simulink model "Main_C0_C3"  (R2023a)
settings: Solver=ode15s  StartTime=0.0  StopTime=1  RelTol=1e-3
model workspace (MAT data in the model file):
  C_IVD = 0.05
  E_IVD1 = 2.1
  E_IVD2 = 2.2
  E_IVD3 = 1.1
  E_IVD4 = 1.7
  E_IVD5 = 3.2
  IVD1 : object (value not decoded)
  IVD2 : object (value not decoded)
  IVD3 : object (value not decoded)
  IVD4 : object (value not decoded)
  IVD5 : object (value not decoded)
  eo_color = [1 0 0]
  io_color = [0 1 0]
  longissimus_color = [1 0 1]
  multifidus_color = [0 1 1]
  muscle_radius = 1
  psoas_color = [0 0 1]
  ra_color = [1 1 0.5]
symbols that are objects in the model workspace (value not decoded): IVD1, IVD2, IVD3, IVD4, IVD5
undefined symbols (not defined in the file or in its folder): AbdFlex, E_TLFflex, IAP_activation_AbdFlex, IAP_Pa, LeftAbdominalMuscleForce, LeftBackMuscleForce, LeftTransverse1MuscleForce, LeftTransverse2MuscleForce, RightAbdominalMuscleForce, RightBackMuscleForce, RightTransverse1MuscleForce, RightTransverse2MuscleForce, TLFflex2, X, Y, Z
libraries: nesl_utility x1235, sm_lib x960, fl_lib x6, simulink_extras x2
(part 6 of 37)

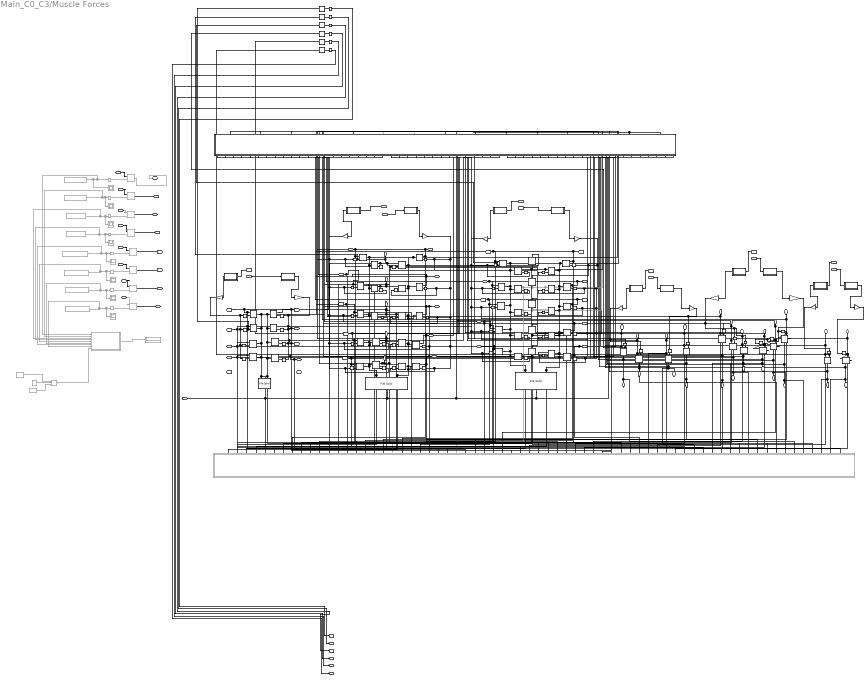
== system Main_C0_C3/Muscle Forces ==
  note: Psoas
  note: Multifidus
  note: Longissimus Thoracis
  note: External Oblique
  note: Internal Oblique
  note: Rectus Abdominus
  note: OldMuscleForces-OBSOLETE
  "Right Psoas " : Inport
  Left Psoas : Inport  Port=2
  "Right MF " : Inport  Port=3
  "Left MF " : Inport  Port=4
  "Right LongThor " : Inport  Port=5
  "Left LongThor " : Inport  Port=6
  "Right EO " : Inport  Port=7
  "Left EO " : Inport  Port=8
  "Right IO " : Inport  Port=9
  "Left IO " : Inport  Port=10
  "Right RA " : Inport  Port=11
  "Left RA " : Inport  Port=12
  Area in mm^2 : Constant  Commented=on  Value=26819
  Constant : Constant  Commented=on  Value=100000
  Display : Display  Commented=on
  Divide : Product  Commented=on  Inputs=**/
  DummyRigid Transform{,1..4} (5 alike) : sm_lib/Frames and Transforms/Rigid Transform  TranslationMethod=None  TranslationStandardOffset=0  TranslationStandardOffsetUnits=m  TranslationStandardAxis=+Z  TranslationCartesianOffset=[0 0 0]  TranslationCartesianOffsetUnits=m  TranslationROffset=0  TranslationROffsetUnits=m  TranslationZOffset=0  TranslationZOffsetUnits=m  TranslationThetaOffset=0  TranslationThetaOffsetUnits=deg  RotationMethod=None  RotationAngleUnits=deg  RotationStandardAxis=+Z  RotationAngle=0.0  RotationArbitraryAxis=[0 0 1]  FollAlignAxisA=+X  BaseAlignAxisA=+Y  FollAlignAxisB=+Y  BaseAlignAxisB=+Z  RotationSequenceAxes=FollowerAxes  RotationSequence=XYX  RotationSequenceAngles=[0 0 0]  RotationSequenceAnglesUnits=deg  RotationMatrix=[1 0 0; 0 1 0; 0 0 1]  Quaternion=[1 0 0 0]
  Gain : Gain  Gain=-0.25
  Gain1 : Gain  Gain=-0.25
  Gain10 : Gain  Gain=-1
  Gain11 : Gain  Gain=-1
  Gain{2..5} (4 alike) : Gain  Gain=-0.1
  Gain6 : Gain  Gain=-0.5
  Gain7 : Gain  Gain=-0.5
  Gain8 : Gain  Gain=-0.3333
  Gain9 : Gain  Gain=-0.3333
  IAP in Pascals : Constant  Commented=on  Value=IAP_Pa
  Internal Force{,1..7} (8 alike) : sm_lib/Forces and Torques/Internal Force  Commented=on
  Internal Force{8..12,14..16,18..69} (60 alike) : sm_lib/Forces and Torques/Internal Force
  Left Abdominal Muscle Force : Constant  Commented=on  Value=-LeftAbdominalMuscleForce
  Left Back Muscle Force : Constant  Commented=on  Value=-LeftBackMuscleForce
  Left Transverse1 Muscle Force : Constant  Commented=on  Value=-LeftTransverse1MuscleForce
  Left Transverse2 Muscle Force : Constant  Commented=on  Value=-LeftTransverse2MuscleForce
  LongissimusThoracis : sm_lib/Body Elements/File Solid  ExtGeomFileName=C:\Users\siril\OneDrive\Desktop\TIM-Control\Matlab\Simscape models\Reduced Order Model\CAD\model without nucleus\LongissimusThoracis.step  UnitType=FromFile  ExtGeomFileUnits=m  StepReaderType=HEX  ExportConvexHullGeometry=off  InertiaType=CalculateFromGeometry  Mass=1  MassUnits=g  CenterOfMass=[0 0 0]  CenterOfMassUnits=m  MomentsOfInertia=[1 1 1]  MomentsOfInertiaUnits=kg*m^2  ProductsOfInertia=[0 0 0]  ProductsOfInertiaUnits=kg*m^2  BasedOnType=Mass  Density=1000  DensityUnits=kg/m^3  DoExposeReferenceFrame=on  SerializedFrames=<Frames><Frame><Id>Frame1</Id><Value><Name>LongissimusThoracis_Right_End</Name><Origin><Source>GeometricFeature</Source><FeatureName>point 13005</FeatureName></Origin><PrimaryAxis><DefinedDirection>+Z</DefinedDirection><Source>ReferenceFrame</Source><SourceDirection>+Z</SourceDirection><FeatureName></FeatureName></PrimaryAxis><SecondaryAxis><DefinedDirection>+X</DefinedDirection><Source>ReferenceFrame</Source><SourceDirection>+X</SourceDirection><FeatureName></FeatureName></SecondaryAxis></Value></Frame><Frame><Id>Frame2</Id><Value><Name>LongissimusThoracis_Left_End</Name><Origin><Source>GeometricFeature</Source><FeatureName>point 10040</FeatureName></Origin><PrimaryAxis><DefinedDirection>+Z</DefinedDirection><Source>ReferenceFrame</Source><SourceDirection>+Z</SourceDirection><FeatureName></FeatureName></PrimaryAxis><SecondaryAxis><DefinedDirection>+X</DefinedDirection><Source>ReferenceFrame</Source><SourceDirection>+X</SourceDirection><FeatureName></FeatureName></SecondaryAxis></Value></Frame></Frames>  GraphicType=None  MarkerShape=Sphere  MarkerSize=10  GraphicVisPropType=SimpleVisualProperties  GraphicDiffuseColor=[0.5 0.5 0.5]  GraphicSpecularColor=[0.5 0.5 0.5 1.0]  GraphicAmbientColor=[0.15 0.15 0.15 1.0]  GraphicEmissiveColor=[0.0 0.0 0.0 1.0]  GraphicShininess=75  GraphicOpacity=0.5
  Multifidus : sm_lib/Body Elements/File Solid  ExtGeomFileName=C:\Users\siril\OneDrive\Desktop\TIM-Control\Matlab\Simscape models\Reduced Order Model\CAD\model without nucleus\Multifidus.step  UnitType=FromFile  ExtGeomFileUnits=m  StepReaderType=HEX  ExportConvexHullGeometry=off  InertiaType=CalculateFromGeometry  Mass=1  MassUnits=g  CenterOfMass=[0 0 0]  CenterOfMassUnits=m  MomentsOfInertia=[1 1 1]  MomentsOfInertiaUnits=kg*m^2  ProductsOfInertia=[0 0 0]  ProductsOfInertiaUnits=kg*m^2  BasedOnType=Mass  Density=1000  DensityUnits=kg/m^3  DoExposeReferenceFrame=on  SerializedFrames=<Frames><Frame><Id>Frame1</Id><Value><Name>Multifidus_Right_End</Name><Origin><Source>GeometricFeature</Source><FeatureName>segment 7296</FeatureName></Origin><PrimaryAxis><DefinedDirection>+Z</DefinedDirection><Source>ReferenceFrame</Source><SourceDirection>+Z</SourceDirection><FeatureName></FeatureName></PrimaryAxis><SecondaryAxis><DefinedDirection>+X</DefinedDirection><Source>ReferenceFrame</Source><SourceDirection>+X</SourceDirection><FeatureName></FeatureName></SecondaryAxis></Value></Frame><Frame><Id>Frame2</Id><Value><Name>Multifidus_Left_End</Name><Origin><Source>GeometricFeature</Source><FeatureName>segment 697</FeatureName></Origin><PrimaryAxis><DefinedDirection>+Z</DefinedDirection><Source>ReferenceFrame</Source><SourceDirection>+Z</SourceDirection><FeatureName></FeatureName></PrimaryAxis><SecondaryAxis><DefinedDirection>+X</DefinedDirection><Source>ReferenceFrame</Source><SourceDirection>+X</SourceDirection><FeatureName></FeatureName></SecondaryAxis></Value></Frame></Frames>  GraphicType=None  MarkerShape=Sphere  MarkerSize=10  GraphicVisPropType=SimpleVisualProperties  GraphicDiffuseColor=[0.5 0.5 0.5]  GraphicSpecularColor=[0.5 0.5 0.5 1.0]  GraphicAmbientColor=[0.15 0.15 0.15 1.0]  GraphicEmissiveColor=[0.0 0.0 0.0 1.0]  GraphicShininess=75  GraphicOpacity=0.5
  Muscle Visualization : Subsystem
  PS Gain : fl_lib/Physical Signals/Functions/PS Gain  gain=-4
  PS Gain1 : fl_lib/Physical Signals/Functions/PS Gain  gain=-10
  PS Gain2 : fl_lib/Physical Signals/Functions/PS Gain  gain=-10
  PS Gain3 : fl_lib/Physical Signals/Functions/PS Gain  gain=-2
  PS Gain4 : fl_lib/Physical Signals/Functions/PS Gain  gain=-3
  PS Gain5 : fl_lib/Physical Signals/Functions/PS Gain  gain=-1
  PS-Simulink Converter{,1..5} (6 alike) : nesl_utility/PS-Simulink Converter  PhysicalDomain=network_engine_domain  SubClassName=ps_output  LeftPortType=input  RightPortType=output  PseudoPeriodic=off  Frequencies=[]  VectorFormat=inherit  Unit=inherit  AffineConversion=off
  Psoas : sm_lib/Body Elements/File Solid  ExtGeomFileName=C:\Users\siril\OneDrive\Desktop\TIM-Control\Matlab\Simscape models\Reduced Order Model\CAD\model without nucleus\Psoas.step  UnitType=FromFile  ExtGeomFileUnits=m  StepReaderType=HEX  ExportConvexHullGeometry=off  InertiaType=CalculateFromGeometry  Mass=1  MassUnits=g  CenterOfMass=[0 0 0]  CenterOfMassUnits=m  MomentsOfInertia=[1 1 1]  MomentsOfInertiaUnits=kg*m^2  ProductsOfInertia=[0 0 0]  ProductsOfInertiaUnits=kg*m^2  BasedOnType=Mass  Density=1000  DensityUnits=kg/m^3  DoExposeReferenceFrame=on  SerializedFrames=<Frames><Frame><Id>Frame1</Id><Value><Name>Psoas_Right_End</Name><Origin><Source>GeometricFeature</Source><FeatureName>point 2042</FeatureName></Origin><PrimaryAxis><DefinedDirection>+Z</DefinedDirection><Source>ReferenceFrame</Source><SourceDirection>+Z</SourceDirection><FeatureName></FeatureName></PrimaryAxis><SecondaryAxis><DefinedDirection>+X</DefinedDirection><Source>ReferenceFrame</Source><SourceDirection>+X</SourceDirection><FeatureName></FeatureName></SecondaryAxis></Value></Frame><Frame><Id>Frame2</Id><Value><Name>Psoas_Left_End</Name><Origin><Source>GeometricFeature</Source><FeatureName>point 14414</FeatureName></Origin><PrimaryAxis><DefinedDirection>+Z</DefinedDirection><Source>ReferenceFrame</Source><SourceDirection>+Z</SourceDirection><FeatureName></FeatureName></PrimaryAxis><SecondaryAxis><DefinedDirection>+X</DefinedDirection><Source>ReferenceFrame</Source><SourceDirection>+X</SourceDirection><FeatureName></FeatureName></SecondaryAxis></Value></Frame></Frames>  GraphicType=None  MarkerShape=Sphere  MarkerSize=10  GraphicVisPropType=SimpleVisualProperties  GraphicDiffuseColor=[0.5 0.5 0.5]  GraphicSpecularColor=[0.5 0.5 0.5 1.0]  GraphicAmbientColor=[0.15 0.15 0.15 1.0]  GraphicEmissiveColor=[0.0 0.0 0.0 1.0]  GraphicShininess=75  GraphicOpacity=0.5
  Right Abdominal Muscle Force : Constant  Commented=on  Value=-RightAbdominalMuscleForce
  Right Back Muscle Force : Constant  Commented=on  Value=-RightBackMuscleForce
  Right Transverse1 Muscle Force : Constant  Commented=on  Value=-RightTransverse1MuscleForce
  Right Transverse2 Muscle Force : Constant  Commented=on  Value=-RightTransverse2MuscleForce
  Scope{1..8} (8 alike) : Scope  Commented=on
  Simulink-PS Converter{,9..12,14..16,18..69} (60 alike) : nesl_utility/Simulink-PS Converter  PhysicalDomain=network_engine_domain  SubClassName=ps_input  LeftPortType=input  RightPortType=output  PseudoPeriodic=off  Frequencies=[]  NoiseDistribution=none  NoiseParameters=[]  Unit=1  AffineConversion=off  FilteringAndDerivatives=provide  SimscapeFilterOrder=1  InputFilterTimeConstant=0.001  UdotUserProvided=0
  Simulink-PS Converter{1..8} (8 alike) : nesl_utility/Simulink-PS Converter  Commented=on  PhysicalDomain=network_engine_domain  SubClassName=ps_input  LeftPortType=input  RightPortType=output  PseudoPeriodic=off  Frequencies=[]  NoiseDistribution=none  NoiseParameters=[]  Unit=1  AffineConversion=off  FilteringAndDerivatives=provide  SimscapeFilterOrder=1  InputFilterTimeConstant=0.001  UdotUserProvided=0
  Subsystem : Subsystem
  Subsystem1 : Subsystem
  Subsystem10 : Subsystem
  Subsystem11 : Subsystem
  Subsystem2 : Subsystem
  Subsystem3 : Subsystem
  Subsystem4 : Subsystem
  Subsystem5 : Subsystem
  Subsystem6 : Subsystem
  Subsystem7 : Subsystem
  Subsystem8 : Subsystem
  Subsystem9 : Subsystem
  Sum of Square of Forces : MATLAB Function  Commented=on  TreatAsAtomicUnit=on
  Visualization : Subsystem  Commented=on
  To Right Abd Muscle on RTS : PMIOPort  Side=Right
  To Right Back Muscle on RTS : PMIOPort  Port=2  Side=Right
  To Right Tr2 Muscle on RTS : PMIOPort  Port=3  Side=Right
  To Right Tr1 Muscle on RTS : PMIOPort  Port=4  Side=Right
  To Left Abd Muscle on S1 : PMIOPort  Port=5  Side=Left
  To Right Abd Muscle on S1 : PMIOPort  Port=6  Side=Left
  To Left Back Muscle on S1 : PMIOPort  Port=7  Side=Left
  To Right Back Muscle on S1 : PMIOPort  Port=8  Side=Left
  To Right Tr2 Muscle on S1 : PMIOPort  Port=9  Side=Left
  To Right Tr1 Muscle on S1 : PMIOPort  Port=10  Side=Left
  To Left Tr2 Muscle on S1 : PMIOPort  Port=11  Side=Left
  To Left Tr1 Muscle on S1 : PMIOPort  Port=12  Side=Left
  To Left Abd Muscle on LTS : PMIOPort  Port=13  Side=Right
  To Left Back Muscle on LTS : PMIOPort  Port=14  Side=Right
  To Left Tr1 Muscle on LTS : PMIOPort  Port=15  Side=Right
  To Left Tr2 Muscle on LTS : PMIOPort  Port=16  Side=Right
  To Origin : PMIOPort  Port=17  Side=Left
  To Psoas_Right_Start_onL1 : PMIOPort  Port=18  Side=Left
  To Psoas_Left_Start_onL1 : PMIOPort  Port=19  Side=Left
  To Psoas_Right_Start_onL2 : PMIOPort  Port=20  Side=Left
  To Psoas_Right_Start_onL3 : PMIOPort  Port=21  Side=Left
  To Psoas_Right_Start_onL4 : PMIOPort  Port=22  Side=Left
  To Psoas_Right_Start_onL5 : PMIOPort  Port=23  Side=Left
  To Psoas_Left_Start_onL2 : PMIOPort  Port=24  Side=Left
  To Psoas_Left_Start_onL3 : PMIOPort  Port=25  Side=Left
  To Psoas_Left_Start_onL4 : PMIOPort  Port=26  Side=Left
  To Psoas_Left_Start_onL5 : PMIOPort  Port=27  Side=Left
  ToMuscles_SpinousProc_onL1 : PMIOPort  Port=28  Side=Left
  ToMuscles_Right_FacetJoint_onL1 : PMIOPort  Port=29  Side=Left
  ToMuscles_Left_FacetJoint_onL1 : PMIOPort  Port=30  Side=Left
  ToMuscles_Right_FacetJoint_onL2 : PMIOPort  Port=31  Side=Left
  ToMuscles_Left_FacetJoint_onL2 : PMIOPort  Port=32  Side=Left
  ToMuscles_SpinousProc_onL2 : PMIOPort  Port=33  Side=Left
  ToMuscles_Right_FacetJoint_onL3 : PMIOPort  Port=34  Side=Left
  ToMuscles_SpinousProc_onL3 : PMIOPort  Port=35  Side=Left
  ToMuscles_Left_FacetJoint_onL3 : PMIOPort  Port=36  Side=Left
  ToMuscles_Right_FacetJoint_onL4 : PMIOPort  Port=37  Side=Left
  ToMuscles_SpinousProc_onL4 : PMIOPort  Port=38  Side=Left
  ToMuscles_Left_FacetJoint_onL4 : PMIOPort  Port=39  Side=Left
  ToMuscles_Right_FacetJoint_onL5 : PMIOPort  Port=40  Side=Left
  ToMuscles_SpinousProc_onL5 : PMIOPort  Port=41  Side=Left
  ToMuscles_Left_FacetJoint_onL5 : PMIOPort  Port=42  Side=Left
  ToMuscles_Right_TransvProc_onL1 : PMIOPort  Port=43  Side=Left
  ToMuscles_Left_TransvProc_onL1 : PMIOPort  Port=44  Side=Left
  ToMuscles_Right_TransvProc_onL2 : PMIOPort  Port=45  Side=Left
  ToMuscles_Right_TransvProc_onL3 : PMIOPort  Port=46  Side=Left
  ToMuscles_Right_TransvProc_onL4 : PMIOPort  Port=47  Side=Left
  ToMuscles_Right_TransvProc_onL5 : PMIOPort  Port=48  Side=Left
  ToMuscles_Left_TransvProc_onL2 : PMIOPort  Port=49  Side=Left
  ToMuscles_Left_TransvProc_onL3 : PMIOPort  Port=50  Side=Left
  ToMuscles_Left_TransvProc_onL4 : PMIOPort  Port=51  Side=Left
  ToMuscles_Left_TransvProc_onL5 : PMIOPort  Port=52  Side=Left
  E01_Right_End_onTSpine : PMIOPort  Port=53  Side=Left
  E01_Left_End_onTSpine : PMIOPort  Port=54  Side=Left
  E02_Right_End_onTSpine : PMIOPort  Port=55  Side=Left
  E02_Left_End_onTSpine : PMIOPort  Port=56  Side=Left
  E01_Right_Start_onS1 : PMIOPort  Port=57  Side=Left
  E02_Right_Start_onS1 : PMIOPort  Port=58  Side=Left
  E01_Left_Start_onS1 : PMIOPort  Port=59  Side=Left
  E02_Left_Start_onS1 : PMIOPort  Port=60  Side=Left
  IO1_Right_End_onTSpine : PMIOPort  Port=61  Side=Left
  IO2_Right_End_onTSpine : PMIOPort  Port=62  Side=Left
  IO3_Right_End_onTSpine : PMIOPort  Port=63  Side=Left
  IO1_Left_End_onTSpine : PMIOPort  Port=64  Side=Left
  IO2_Left_End_onTSpine : PMIOPort  Port=65  Side=Left
  IO3_Left_End_onTSpine : PMIOPort  Port=66  Side=Left
  IO1_Right_Start_onS1 : PMIOPort  Port=67  Side=Left
  IO2_Right_Start_onS1 : PMIOPort  Port=68  Side=Left
  IO3_Right_Start_onS1 : PMIOPort  Port=69  Side=Left
  IO1_Left_Start_onS1 : PMIOPort  Port=70  Side=Left
  IO2_Left_Start_onS1 : PMIOPort  Port=71  Side=Left
  IO3_Left_Start_onS1 : PMIOPort  Port=72  Side=Left
  RA_Right_End_onTSpine : PMIOPort  Port=73  Side=Left
  RA_Left_End_onTSpine : PMIOPort  Port=74  Side=Left
  RA_Right_Start_onS1 : PMIOPort  Port=75  Side=Left
  RA_Left_Start_onS1 : PMIOPort  Port=76  Side=Left
  Left Psoas force : Outport
  Left MF force : Outport  Port=2
  Left LongThor force : Outport  Port=3
  Left EO force : Outport  Port=4
  Left IO force : Outport  Port=5
  Left RA force : Outport  Port=6
  wires:
  "Left RA "/1 -> Subsystem11/1(Muslce force)
  "Right RA "/1 -> Subsystem10/1(Muslce force)
  "Left IO "/1 -> Subsystem9/1(Muslce force)
  "Right IO "/1 -> Subsystem8/1(Muslce force)
  "Left EO "/1 -> Subsystem7/1(Muslce force)
  "Right EO "/1 -> Subsystem6/1(Muslce force)
  "Left LongThor "/1 -> Subsystem5/1(Muslce force)
  "Right LongThor "/1 -> Subsystem4/1(Muslce force)
  "Left MF "/1 -> Subsystem3/1(Muslce force)
  "Right MF "/1 -> Subsystem2/1(Muslce force)
  Left Psoas/1 -> Subsystem1/1(Muslce force)
  "Right Psoas "/1 -> Subsystem/1(Muslce force)
  PS-Simulink Converter5/1 -> Left RA force/1  "Left RA"
  PS-Simulink Converter4/1 -> Left IO force/1  "Left IO"
  PS-Simulink Converter3/1 -> Left EO force/1  "Left EO"
  PS-Simulink Converter2/1 -> Left LongThor force/1  "Left LongThor"
  PS-Simulink Converter1/1 -> Left MF force/1  "Left MF"
  PS-Simulink Converter/1 -> Left Psoas force/1  "Left Psoas"
  Subsystem11/1(Out1) -> Gain11/1
  Subsystem10/1(Out1) -> Gain10/1
  Subsystem9/1(Out1) -> Gain9/1
  Subsystem8/1(Out1) -> Gain8/1
  Subsystem7/1(Out1) -> Gain6/1
  Subsystem6/1(Out1) -> Gain7/1
  Subsystem5/1(Out1) -> Gain4/1
  Subsystem4/1(Out1) -> Gain5/1
  Subsystem3/1(Out1) -> Gain3/1
  Subsystem2/1(Out1) -> Gain2/1
  Gain11/1 -> Simulink-PS Converter69/1
  Gain10/1 -> Simulink-PS Converter68/1
  Subsystem1/1(Out1) -> Gain1/1
  Subsystem/1(Out1) -> Gain/1
  Gain9/1 -> Simulink-PS Converter67/1, Simulink-PS Converter66/1, Simulink-PS Converter65/1
  Gain8/1 -> Simulink-PS Converter64/1, Simulink-PS Converter63/1, Simulink-PS Converter62/1
  Gain7/1 -> Simulink-PS Converter59/1, Simulink-PS Converter58/1
  Gain6/1 -> Simulink-PS Converter60/1, Simulink-PS Converter61/1
  Gain4/1 -> Simulink-PS Converter40/1, Simulink-PS Converter41/1, Simulink-PS Converter44/1, Simulink-PS Converter45/1, Simulink-PS Converter49/1, Simulink-PS Converter47/1, Simulink-PS Converter52/1, Simulink-PS Converter51/1, Simulink-PS Converter56/1, Simulink-PS Converter55/1
  Gain5/1 -> Simulink-PS Converter42/1, Simulink-PS Converter43/1, Simulink-PS Converter46/1, Simulink-PS Converter48/1, Simulink-PS Converter50/1, Simulink-PS Converter53/1, Simulink-PS Converter54/1, Simulink-PS Converter57/1, Simulink-PS Converter38/1, Simulink-PS Converter39/1
  Gain3/1 -> Simulink-PS Converter25/1, Simulink-PS Converter24/1, Simulink-PS Converter29/1, Simulink-PS Converter28/1, Simulink-PS Converter33/1, Simulink-PS Converter32/1, Simulink-PS Converter37/1, Simulink-PS Converter36/1, Simulink-PS Converter19/1, Simulink-PS Converter21/1
  Gain2/1 -> Simulink-PS Converter26/1, Simulink-PS Converter27/1, Simulink-PS Converter30/1, Simulink-PS Converter31/1, Simulink-PS Converter34/1, Simulink-PS Converter35/1, Simulink-PS Converter22/1, Simulink-PS Converter23/1, Simulink-PS Converter20/1, Simulink-PS Converter18/1
  Gain1/1 -> Simulink-PS Converter16/1, Simulink-PS Converter15/1, Simulink-PS Converter14/1, Simulink-PS Converter9/1
  Gain/1 -> Simulink-PS Converter/1, Simulink-PS Converter10/1, Simulink-PS Converter11/1, Simulink-PS Converter12/1
  Divide/1 -> Sum of Square of Forces/9(IAP)
  Area in mm^2/1 -> Divide/2
  Constant/1 -> Divide/3
  IAP in Pascals/1 -> Divide/1
  Left Transverse2 Muscle Force/1 -> Simulink-PS Converter8/1, Scope8/1, Sum of Square of Forces/8(F8)  "LeftTransverse2MuscleForce"
  Right Transverse1 Muscle Force/1 -> Sum of Square of Forces/7(F7), Simulink-PS Converter5/1, Scope5/1  "RightTransverse1MuscleForce"
  Left Transverse1 Muscle Force/1 -> Sum of Square of Forces/6(F6), Simulink-PS Converter7/1, Scope7/1  "LeftTransverse1MuscleForce"
  Right Transverse2 Muscle Force/1 -> Simulink-PS Converter6/1, Scope6/1, Sum of Square of Forces/5(F5)  "RightTransverse2MuscleForce"
  Left Back Muscle Force/1 -> Simulink-PS Converter4/1, Scope4/1, Sum of Square of Forces/4(F4)  "LeftBackMuscleForce"
  Right Back Muscle Force/1 -> Sum of Square of Forces/3(F3), Simulink-PS Converter3/1, Scope3/1  "RightBackMuscleForce"
  Left Abdominal Muscle Force/1 -> Sum of Square of Forces/2(F2), Simulink-PS Converter2/1, Scope2/1  "LeftAbdominalMuscleForce"
  Right Abdominal Muscle Force/1 -> Scope1/1, Simulink-PS Converter1/1, Sum of Square of Forces/1(F1)  "RightAbdominalMuscleForce"
  Sum of Square of Forces/1(SumofSquareofForces) -> Display/1  "SumofSquareofForces"
  connections:
  PS-Simulink Converter5/LConn1 -- PS Gain5/RConn1
  PS-Simulink Converter4/LConn1 -- PS Gain4/RConn1
  PS-Simulink Converter3/LConn1 -- PS Gain3/RConn1
  PS-Simulink Converter2/LConn1 -- PS Gain2/RConn1
  PS-Simulink Converter1/LConn1 -- PS Gain1/RConn1
  PS-Simulink Converter/LConn1 -- PS Gain/RConn1
  Muscle Visualization/RConn56 -- Psoas/RConn1 -- To Origin/RConn1 -- Multifidus/RConn1 -- Muscle Visualization/LConn14 -- Muscle Visualization/LConn15 -- LongissimusThoracis/RConn1
  Multifidus/LConn1 -- Visualization/LConn2 -- Internal Force34/RConn1 -- Internal Force35/RConn1 -- Internal Force30/RConn1 -- Internal Force27/RConn1 -- Internal Force26/RConn1 -- Internal Force23/RConn1 -- Internal Force22/RConn1 -- Internal Force19/RConn1 -- Internal Force18/RConn1 -- Muscle Visualization/LConn1 -- Internal Force31/RConn1
  ToMuscles_SpinousProc_onL1/RConn1 -- Muscle Visualization/RConn5 -- Internal Force20/LConn1 -- DummyRigid Transform/LConn1 -- Visualization/LConn12 -- Internal Force19/LConn1
  ToMuscles_Left_FacetJoint_onL4/RConn1 -- Muscle Visualization/RConn29 -- Internal Force33/LConn1 -- Visualization/LConn37
  IO3_Left_End_onTSpine/RConn1 -- Muscle Visualization/RConn19 -- Visualization/LConn28 -- Internal Force67/LConn1
  RA_Right_End_onTSpine/RConn1 -- Muscle Visualization/RConn36 -- Visualization/LConn48 -- Internal Force68/LConn1
  DummyRigid Transform3/RConn1 -- Visualization/LConn38 -- Internal Force51/LConn1 -- Muscle Visualization/LConn10 -- Internal Force53/LConn1
  LongissimusThoracis/LConn1 -- Visualization/LConn3 -- Internal Force57/RConn1 -- Internal Force54/RConn1 -- Internal Force39/RConn1 -- Muscle Visualization/LConn3 -- Internal Force38/RConn1 -- Internal Force42/RConn1 -- Internal Force43/RConn1 -- Internal Force46/RConn1 -- Internal Force48/RConn1 -- Internal Force50/RConn1 -- Internal Force53/RConn1
  Internal Force69/RConn1 -- Muscle Visualization/RConn54 -- Visualization/LConn67 -- RA_Left_Start_onS1/RConn1
  Internal Force68/RConn1 -- Muscle Visualization/RConn55 -- Visualization/LConn66 -- RA_Right_Start_onS1/RConn1
  RA_Left_End_onTSpine/RConn1 -- Muscle Visualization/RConn32 -- Visualization/LConn50 -- Internal Force69/LConn1
  Simulink-PS Converter69/RConn1 -- Internal Force69/LConn2
  Internal Force68/LConn2 -- PS Gain5/LConn1 -- Simulink-PS Converter68/RConn1
  Internal Force67/RConn1 -- Muscle Visualization/RConn51 -- Visualization/LConn64 -- IO3_Left_Start_onS1/RConn1
  IO2_Left_End_onTSpine/RConn1 -- Muscle Visualization/RConn25 -- Visualization/LConn31 -- Internal Force66/LConn1
  Internal Force66/RConn1 -- Muscle Visualization/RConn49 -- Visualization/LConn62 -- IO2_Left_Start_onS1/RConn1
  IO1_Left_End_onTSpine/RConn1 -- Muscle Visualization/RConn30 -- Visualization/LConn40 -- Internal Force65/LConn1
  Internal Force65/RConn1 -- Muscle Visualization/RConn47 -- Visualization/LConn56 -- IO1_Left_Start_onS1/RConn1
  IO3_Right_End_onTSpine/RConn1 -- Muscle Visualization/RConn18 -- Visualization/LConn34 -- Internal Force64/LConn1
  Internal Force64/RConn1 -- Muscle Visualization/RConn40 -- Visualization/LConn68 -- IO3_Right_Start_onS1/RConn1
  IO2_Right_End_onTSpine/RConn1 -- Muscle Visualization/RConn24 -- Visualization/LConn36 -- Internal Force63/LConn1
  Internal Force63/RConn1 -- Muscle Visualization/RConn45 -- Visualization/LConn58 -- IO2_Right_Start_onS1/RConn1
  Internal Force62/RConn1 -- Muscle Visualization/RConn43 -- Visualization/LConn54 -- IO1_Right_Start_onS1/RConn1
  Internal Force62/LConn1 -- Visualization/LConn41 -- Muscle Visualization/RConn31 -- IO1_Right_End_onTSpine/RConn1
  Simulink-PS Converter67/RConn1 -- Internal Force67/LConn2
  Simulink-PS Converter65/RConn1 -- Internal Force65/LConn2
  Simulink-PS Converter66/RConn1 -- Internal Force66/LConn2
  Internal Force64/LConn2 -- PS Gain4/LConn1 -- Simulink-PS Converter64/RConn1
  Simulink-PS Converter63/RConn1 -- Internal Force63/LConn2
  Simulink-PS Converter62/RConn1 -- Internal Force62/LConn2
  E02_Left_End_onTSpine/RConn1 -- Muscle Visualization/RConn27 -- Visualization/LConn39 -- Internal Force61/LConn1
  E02_Left_Start_onS1/RConn1 -- Visualization/LConn18 -- Muscle Visualization/RConn50 -- Internal Force61/RConn1
  E01_Left_End_onTSpine/RConn1 -- Muscle Visualization/RConn35 -- Visualization/LConn47 -- Internal Force60/LConn1
  Internal Force60/RConn1 -- Muscle Visualization/RConn52 -- Visualization/LConn60 -- E01_Left_Start_onS1/RConn1
  Internal Force58/LConn1 -- Visualization/LConn49 -- Muscle Visualization/RConn34 -- E01_Right_End_onTSpine/RConn1
  E02_Right_Start_onS1/RConn1 -- Visualization/LConn63 -- Muscle Visualization/RConn48 -- Internal Force59/RConn1
  Internal Force59/LConn1 -- Visualization/LConn42 -- Muscle Visualization/RConn26 -- E02_Right_End_onTSpine/RConn1
  E01_Right_Start_onS1/RConn1 -- Visualization/LConn61 -- Muscle Visualization/RConn53 -- Internal Force58/RConn1
  Simulink-PS Converter61/RConn1 -- Internal Force61/LConn2
  Simulink-PS Converter60/RConn1 -- Internal Force60/LConn2
  Internal Force59/LConn2 -- PS Gain3/LConn1 -- Simulink-PS Converter59/RConn1
  Simulink-PS Converter58/RConn1 -- Internal Force58/LConn2
  ToMuscles_Left_TransvProc_onL5/RConn1 -- Muscle Visualization/RConn39 -- Visualization/LConn46 -- Internal Force56/LConn1
  DummyRigid Transform4/RConn1 -- Visualization/LConn52 -- Internal Force55/LConn1 -- Muscle Visualization/LConn12 -- Internal Force57/LConn1
  Internal Force54/LConn1 -- Visualization/LConn45 -- Muscle Visualization/RConn38 -- ToMuscles_Right_TransvProc_onL5/RConn1
  Simulink-PS Converter57/RConn1 -- Internal Force57/LConn2
  Simulink-PS Converter56/RConn1 -- Internal Force56/LConn2
  Simulink-PS Converter55/RConn1 -- Internal Force55/LConn2
  Simulink-PS Converter54/RConn1 -- Internal Force54/LConn2
  ToMuscles_Left_TransvProc_onL4/RConn1 -- Muscle Visualization/RConn21 -- Visualization/LConn29 -- Internal Force52/LConn1
  Internal Force50/LConn1 -- Visualization/LConn30 -- Muscle Visualization/RConn20 -- ToMuscles_Right_TransvProc_onL4/RConn1
  Simulink-PS Converter53/RConn1 -- Internal Force53/LConn2
  Simulink-PS Converter52/RConn1 -- Internal Force52/LConn2
  Simulink-PS Converter51/RConn1 -- Internal Force51/LConn2
  Simulink-PS Converter50/RConn1 -- Internal Force50/LConn2
  ToMuscles_Left_TransvProc_onL3/RConn1 -- Muscle Visualization/RConn12 -- Visualization/LConn20 -- Internal Force49/LConn1
  Visualization/LConn26 -- DummyRigid Transform2/RConn1 -- Internal Force47/LConn1 -- Muscle Visualization/LConn7 -- Internal Force48/LConn1
  Internal Force46/LConn1 -- Visualization/LConn22 -- Muscle Visualization/RConn11 -- ToMuscles_Right_TransvProc_onL3/RConn1
  Simulink-PS Converter49/RConn1 -- Internal Force49/LConn2
  Simulink-PS Converter48/RConn1 -- Internal Force48/LConn2
  Simulink-PS Converter47/RConn1 -- Internal Force47/LConn2
  Simulink-PS Converter46/RConn1 -- Internal Force46/LConn2
  ToMuscles_Left_TransvProc_onL2/RConn1 -- Muscle Visualization/RConn9 -- Visualization/LConn16 -- Internal Force44/LConn1
  Visualization/LConn19 -- DummyRigid Transform1/RConn1 -- Internal Force45/LConn1 -- Muscle Visualization/LConn6 -- Internal Force43/LConn1
  Internal Force42/LConn1 -- Visualization/LConn15 -- Muscle Visualization/RConn8 -- ToMuscles_Right_TransvProc_onL2/RConn1
  Simulink-PS Converter45/RConn1 -- Internal Force45/LConn2
  Simulink-PS Converter44/RConn1 -- Internal Force44/LConn2
  Simulink-PS Converter43/RConn1 -- Internal Force43/LConn2
  Simulink-PS Converter42/RConn1 -- Internal Force42/LConn2
  Internal Force39/LConn1 -- Visualization/LConn7 -- Internal Force41/LConn1 -- Muscle Visualization/LConn5 -- DummyRigid Transform/RConn1
  LongissimusThoracis/LConn2 -- Visualization/LConn4 -- Internal Force56/RConn1 -- Internal Force55/RConn1 -- Internal Force51/RConn1 -- Internal Force52/RConn1 -- Internal Force47/RConn1 -- Internal Force49/RConn1 -- Internal Force45/RConn1 -- Internal Force44/RConn1 -- Internal Force41/RConn1 -- Muscle Visualization/LConn4 -- Internal Force40/RConn1
  Internal Force40/LConn1 -- Visualization/LConn9 -- Muscle Visualization/RConn4 -- ToMuscles_Left_TransvProc_onL1/RConn1
  Internal Force38/LConn1 -- Visualization/LConn11 -- Muscle Visualization/RConn3 -- ToMuscles_Right_TransvProc_onL1/RConn1
  Simulink-PS Converter41/RConn1 -- Internal Force41/LConn2
  Simulink-PS Converter40/RConn1 -- Internal Force40/LConn2
  Simulink-PS Converter39/RConn1 -- Internal Force39/LConn2
  Internal Force38/LConn2 -- PS Gain2/LConn1 -- Simulink-PS Converter38/RConn1
  ToMuscles_SpinousProc_onL5/RConn1 -- DummyRigid Transform4/LConn1 -- Visualization/LConn57 -- Internal Force36/LConn1 -- Muscle Visualization/LConn13 -- Internal Force35/LConn1
  Internal Force37/LConn1 -- Visualization/LConn59 -- Muscle Visualization/RConn42 -- ToMuscles_Left_FacetJoint_onL5/RConn1
  Internal Force34/LConn1 -- Visualization/LConn53 -- Muscle Visualization/RConn46 -- ToMuscles_Right_FacetJoint_onL5/RConn1
  Simulink-PS Converter37/RConn1 -- Internal Force37/LConn2
  Simulink-PS Converter36/RConn1 -- Internal Force36/LConn2
  Simulink-PS Converter35/RConn1 -- Internal Force35/LConn2
  Simulink-PS Converter34/RConn1 -- Internal Force34/LConn2
  ToMuscles_SpinousProc_onL4/RConn1 -- Muscle Visualization/LConn11 -- DummyRigid Transform3/LConn1 -- Visualization/LConn6 -- Internal Force32/LConn1 -- Internal Force31/LConn1
  Internal Force30/LConn1 -- Visualization/LConn35 -- Muscle Visualization/RConn28 -- ToMuscles_Right_FacetJoint_onL4/RConn1
  Simulink-PS Converter33/RConn1 -- Internal Force33/LConn2
  Simulink-PS Converter32/RConn1 -- Internal Force32/LConn2
  Simulink-PS Converter31/RConn1 -- Internal Force31/LConn2
  Simulink-PS Converter30/RConn1 -- Internal Force30/LConn2
  ToMuscles_Left_FacetJoint_onL3/RConn1 -- Visualization/LConn23 -- Muscle Visualization/RConn14 -- Internal Force29/LConn1
  ToMuscles_SpinousProc_onL3/RConn1 -- Muscle Visualization/RConn15 -- DummyRigid Transform2/LConn1 -- Internal Force28/LConn1 -- Visualization/LConn27 -- Internal Force27/LConn1
  Internal Force26/LConn1 -- Visualization/LConn21 -- Muscle Visualization/RConn13 -- ToMuscles_Right_FacetJoint_onL3/RConn1
  Simulink-PS Converter29/RConn1 -- Internal Force29/LConn2
  Simulink-PS Converter28/RConn1 -- Internal Force28/LConn2
  Simulink-PS Converter27/RConn1 -- Internal Force27/LConn2
  Simulink-PS Converter26/RConn1 -- Internal Force26/LConn2
  Internal Force25/LConn1 -- Visualization/LConn14 -- Muscle Visualization/RConn7 -- ToMuscles_Left_FacetJoint_onL2/RConn1
  Internal Force23/LConn1 -- Visualization/LConn17 -- Internal Force24/LConn1 -- Muscle Visualization/RConn10 -- DummyRigid Transform1/LConn1 -- ToMuscles_SpinousProc_onL2/RConn1
  Internal Force22/LConn1 -- Visualization/LConn13 -- Muscle Visualization/RConn6 -- ToMuscles_Right_FacetJoint_onL2/RConn1
  Simulink-PS Converter25/RConn1 -- Internal Force25/LConn2
  Simulink-PS Converter24/RConn1 -- Internal Force24/LConn2
  Simulink-PS Converter23/RConn1 -- Internal Force23/LConn2
  Simulink-PS Converter22/RConn1 -- Internal Force22/LConn2
  Internal Force18/LConn2 -- PS Gain1/LConn1 -- Simulink-PS Converter18/RConn1
  Simulink-PS Converter19/RConn1 -- Internal Force21/LConn2
  Simulink-PS Converter20/RConn1 -- Internal Force19/LConn2
  Simulink-PS Converter21/RConn1 -- Internal Force20/LConn2
  Internal Force28/RConn1 -- Internal Force36/RConn1 -- Multifidus/LConn2 -- Visualization/LConn1 -- Internal Force37/RConn1 -- Internal Force33/RConn1 -- Internal Force32/RConn1 -- Internal Force29/RConn1 -- Internal Force24/RConn1 -- Internal Force25/RConn1 -- Internal Force20/RConn1 -- Muscle Visualization/LConn2 -- Internal Force21/RConn1
  ToMuscles_Left_FacetJoint_onL1/RConn1 -- Muscle Visualization/RConn2 -- Visualization/LConn8 -- Internal Force21/LConn1
  ToMuscles_Right_FacetJoint_onL1/RConn1 -- Muscle Visualization/RConn1 -- Visualization/LConn10 -- Internal Force18/LConn1
  Internal Force16/LConn1 -- Muscle Visualization/RConn41 -- Visualization/LConn55 -- To Psoas_Left_Start_onL4/RConn1
  Internal Force15/LConn1 -- Muscle Visualization/RConn33 -- Visualization/LConn43 -- To Psoas_Left_Start_onL3/RConn1
  Internal Force14/LConn1 -- Muscle Visualization/RConn23 -- Visualization/LConn32 -- To Psoas_Left_Start_onL2/RConn1
  Simulink-PS Converter16/RConn1 -- Internal Force16/LConn2
  Simulink-PS Converter15/RConn1 -- Internal Force15/LConn2
  Simulink-PS Converter14/RConn1 -- Internal Force14/LConn2
  Simulink-PS Converter12/RConn1 -- Internal Force12/LConn2
  Simulink-PS Converter11/RConn1 -- Internal Force11/LConn2
  Internal Force10/LConn2 -- PS Gain/LConn1 -- Simulink-PS Converter10/RConn1
  Internal Force12/LConn1 -- Visualization/LConn51 -- Muscle Visualization/RConn44 -- To Psoas_Right_Start_onL4/RConn1
  Internal Force11/LConn1 -- Visualization/LConn44 -- Muscle Visualization/RConn37 -- To Psoas_Right_Start_onL3/RConn1
  Internal Force10/LConn1 -- Muscle Visualization/RConn22 -- Visualization/LConn33 -- To Psoas_Right_Start_onL2/RConn1
  Simulink-PS Converter9/RConn1 -- Internal Force9/LConn2
  Simulink-PS Converter/RConn1 -- Internal Force8/LConn2
  Psoas/LConn2 -- Visualization/LConn65 -- Internal Force16/RConn1 -- Internal Force15/RConn1 -- Internal Force14/RConn1 -- Muscle Visualization/LConn9 -- Internal Force9/RConn1
  To Psoas_Left_Start_onL1/RConn1 -- Visualization/LConn25 -- Muscle Visualization/RConn17 -- Internal Force9/LConn1
  Internal Force10/RConn1 -- Internal Force11/RConn1 -- Internal Force12/RConn1 -- Psoas/LConn1 -- Visualization/LConn5 -- Muscle Visualization/LConn8 -- Internal Force8/RConn1
  Internal Force8/LConn1 -- Visualization/LConn24 -- Muscle Visualization/RConn16 -- To Psoas_Right_Start_onL1/RConn1
  Internal Force/RConn1 -- To Right Abd Muscle on RTS/RConn1
  To Left Abd Muscle on S1/RConn1 -- Internal Force1/LConn1
  To Left Tr2 Muscle on LTS/RConn1 -- Internal Force7/RConn1
  To Left Tr1 Muscle on S1/RConn1 -- Internal Force6/LConn1
  To Right Tr1 Muscle on S1/RConn1 -- Internal Force4/LConn1
  To Right Tr2 Muscle on S1/RConn1 -- Internal Force5/LConn1
  To Left Back Muscle on LTS/RConn1 -- Internal Force3/RConn1
  Simulink-PS Converter7/RConn1 -- Internal Force6/LConn2
  Simulink-PS Converter5/RConn1 -- Internal Force4/LConn2
  Simulink-PS Converter4/RConn1 -- Internal Force3/LConn2
  To Right Abd Muscle on S1/RConn1 -- Internal Force/LConn1
  Simulink-PS Converter3/RConn1 -- Internal Force2/LConn2
  Simulink-PS Converter2/RConn1 -- Internal Force1/LConn2
  To Left Abd Muscle on LTS/RConn1 -- Internal Force1/RConn1
  To Right Back Muscle on RTS/RConn1 -- Internal Force2/RConn1
  Internal Force7/LConn1 -- To Left Tr2 Muscle on S1/RConn1
  To Right Tr2 Muscle on RTS/RConn1 -- Internal Force5/RConn1
  To Left Tr1 Muscle on LTS/RConn1 -- Internal Force6/RConn1
  Simulink-PS Converter1/RConn1 -- Internal Force/LConn2
  Simulink-PS Converter6/RConn1 -- Internal Force5/LConn2
  To Right Tr1 Muscle on RTS/RConn1 -- Internal Force4/RConn1
  Simulink-PS Converter8/RConn1 -- Internal Force7/LConn2
  To Left Back Muscle on S1/RConn1 -- Internal Force3/LConn1
  Internal Force2/LConn1 -- To Right Back Muscle on S1/RConn1

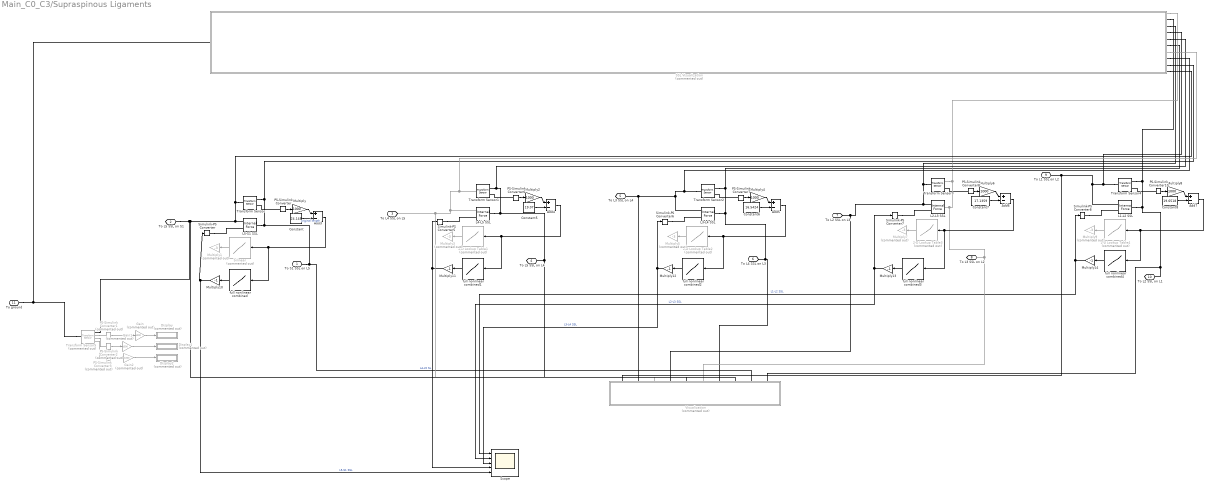
== system Main_C0_C3/Supraspinous Ligaments ==
  2-D Lookup Table1 : Lookup_n-D  Commented=on  NumberOfTableDimensions=1  BreakpointsForDimension1=[0;0.223;3.345;4.906;6.467]  BreakpointsForDimension2=[1:3]  Table=[0;0;8.4;21;84]  InternalRulePriority=Speed  RndMeth=Simplest
  2-D Lookup Table2 : Lookup_n-D  Commented=on  NumberOfTableDimensions=1  BreakpointsForDimension1=[0;0.194;2.91;4.268;5.626]  BreakpointsForDimension2=[1:3]  Table=[0;0;8.4;21;84]  InternalRulePriority=Speed  RndMeth=Simplest
  2-D Lookup Table3 : Lookup_n-D  Commented=on  NumberOfTableDimensions=1  BreakpointsForDimension1=[0;0.268;4.02;5.896;7.772]  BreakpointsForDimension2=[1:3]  Table=[0;0;8.4;21;84]  InternalRulePriority=Speed  RndMeth=Simplest
  2-D Lookup Table4 : Lookup_n-D  Commented=on  NumberOfTableDimensions=1  BreakpointsForDimension1=[0;0.223;3.345;4.906;6.467]  BreakpointsForDimension2=[1:3]  Table=[0;0;8.4;21;84]  InternalRulePriority=Speed  RndMeth=Simplest
  Add{3..7} (5 alike) : Sum  Inputs=+-
  Constant : Constant  Value=24.148
  Constant5 : Constant  Value=19.07
  Constant6 : Constant  Value=16.5424
  Constant7 : Constant  Value=17.1359
  Constant8 : Constant  Value=19.6518
  Display : Display  Commented=on
  Display1 : Display  Commented=on
  Display2 : Display  Commented=on
  Gain : Gain  Commented=on  Gain=1000
  Gain1 : Gain  Commented=on  Gain=1000
  Gain2 : Gain  Commented=on  Gain=1000
  L1-L2 SSL : sm_lib/Forces and Torques/Internal Force
  L2-L3 SSL : sm_lib/Forces and Torques/Internal Force
  L3-L4 SSL : sm_lib/Forces and Torques/Internal Force
  L4-L5 SSL : sm_lib/Forces and Torques/Internal Force
  L5-S1 SSL : sm_lib/Forces and Torques/Internal Force
  Multiply{,2,4,6,8} (5 alike) : Gain  Gain=1000
  Multiply{1,3,5,7,9} (5 alike) : Gain  Commented=on  Gain=-3
  Multiply{10..14} (5 alike) : Gain  Gain=-1
  PS-Simulink Converter{,6..8,10} (5 alike) : nesl_utility/PS-Simulink Converter  PhysicalDomain=network_engine_domain  SubClassName=ps_output  LeftPortType=input  RightPortType=output  PseudoPeriodic=off  Frequencies=[]  VectorFormat=inherit  Unit=inherit  AffineConversion=off
  PS-Simulink Converter1 : nesl_utility/PS-Simulink Converter  Commented=on  PhysicalDomain=network_engine_domain  SubClassName=ps_output  LeftPortType=input  RightPortType=output  PseudoPeriodic=off  Frequencies=[]  VectorFormat=inherit  Unit=inherit  AffineConversion=off
  PS-Simulink Converter2 : nesl_utility/PS-Simulink Converter  Commented=on  PhysicalDomain=network_engine_domain  SubClassName=ps_output  LeftPortType=input  RightPortType=output  PseudoPeriodic=off  Frequencies=[]  VectorFormat=inherit  Unit=inherit  AffineConversion=off
  PS-Simulink Converter3 : nesl_utility/PS-Simulink Converter  Commented=on  PhysicalDomain=network_engine_domain  SubClassName=ps_output  LeftPortType=input  RightPortType=output  PseudoPeriodic=off  Frequencies=[]  VectorFormat=inherit  Unit=inherit  AffineConversion=off
  SSL Visualization : Subsystem  Commented=on
  Scope : Scope  NumInputPorts=5
  Simulink-PS Converter{,5..8} (5 alike) : nesl_utility/Simulink-PS Converter  PhysicalDomain=network_engine_domain  SubClassName=ps_input  LeftPortType=input  RightPortType=output  PseudoPeriodic=off  Frequencies=[]  NoiseDistribution=none  NoiseParameters=[]  Unit=1  AffineConversion=off  FilteringAndDerivatives=provide  SimscapeFilterOrder=1  InputFilterTimeConstant=0.001  UdotUserProvided=0
  Transform Sensor{,1..4} (5 alike) : sm_lib/Frames and Transforms/Transform Sensor  MeasurementFrame=World  RotationSequence=XYX  SenseAngle=off  SenseAxis=off  SenseQ=off  SenseR=off  SenseRotationSequence=off  SenseOmegaX=off  SenseOmegaY=off  SenseOmegaZ=off  SenseQDot=off  SenseRDot=off  SenseRotationSequenceDot=off  SenseAlphaX=off  SenseAlphaY=off  SenseAlphaZ=off  SenseQDDot=off  SenseRDDot=off  SenseX=off  SenseY=off  SenseZ=off  SenseRad=off  SenseAzim=off  SenseDist=on  SenseInc=off  SenseXDot=off  SenseYDot=off  SenseZDot=off  SenseRadDot=off  SenseAzimDot=off  SenseDistDot=off  SenseIncDot=off  SenseXDDot=off  SenseYDDot=off  SenseZDDot=off  SenseRadDDot=off  SenseAzimDDot=off  SenseDistDDot=off  SenseIncDDot=off
  Transform Sensor5 : sm_lib/Frames and Transforms/Transform Sensor  Commented=on  MeasurementFrame=World  RotationSequence=XYZ  SenseAngle=off  SenseAxis=off  SenseQ=off  SenseR=off  SenseRotationSequence=off  SenseOmegaX=off  SenseOmegaY=off  SenseOmegaZ=off  SenseQDot=off  SenseRDot=off  SenseRotationSequenceDot=off  SenseAlphaX=off  SenseAlphaY=off  SenseAlphaZ=off  SenseQDDot=off  SenseRDDot=off  SenseX=on  SenseY=on  SenseZ=on  SenseRad=off  SenseAzim=off  SenseDist=off  SenseInc=off  SenseXDot=off  SenseYDot=off  SenseZDot=off  SenseRadDot=off  SenseAzimDot=off  SenseDistDot=off  SenseIncDot=off  SenseXDDot=off  SenseYDDot=off  SenseZDDot=off  SenseRadDDot=off  SenseAzimDDot=off  SenseDistDDot=off  SenseIncDDot=off
  Visualization : Subsystem  Commented=on
  bilinear : Lookup_n-D  Commented=on  NumberOfTableDimensions=1  BreakpointsForDimension1=[0;0.272;4.08;5.984;7.888]  BreakpointsForDimension2=[1:3]  Table=[0;0;8.4;21;84]  InternalRulePriority=Speed  RndMeth=Simplest
  full nonlinear combined : Lookup_n-D  NumberOfTableDimensions=1  BreakpointsForDimension1=[0;3.634295;5.301569;5.928566;6.545615;7.122779]  BreakpointsForDimension2=[1:3]  Table=[0;30.51213;75.18927;150.629;224.502;299.8224]  InternalRulePriority=Speed  RndMeth=Simplest
  full nonlinear combined1 : Lookup_n-D  NumberOfTableDimensions=1  BreakpointsForDimension1=[0;2.870052;4.18672;4.681868;5.16916;5.624954]  BreakpointsForDimension2=[1:3]  Table=[0;30.51213;75.18927;150.629;224.502;299.8224]  InternalRulePriority=Speed  RndMeth=Simplest
  full nonlinear combined2 : Lookup_n-D  NumberOfTableDimensions=1  BreakpointsForDimension1=[0;2.489646;3.631798;4.061318;4.484023;4.879404]  BreakpointsForDimension2=[1:3]  Table=[0;30.51213;75.18927;150.629;224.502;299.8224]  InternalRulePriority=Speed  RndMeth=Simplest
  full nonlinear combined3 : Lookup_n-D  NumberOfTableDimensions=1  BreakpointsForDimension1=[0;2.578968;3.762098;4.207028;4.644899;5.054465]  BreakpointsForDimension2=[1:3]  Table=[0;30.51213;75.18927;150.629;224.502;299.8224]  InternalRulePriority=Speed  RndMeth=Simplest
  full nonlinear combined4 : Lookup_n-D  NumberOfTableDimensions=1  BreakpointsForDimension1=[0;2.957613;4.314451;4.824706;5.326864;5.796564]  BreakpointsForDimension2=[1:3]  Table=[0;30.51213;75.18927;150.629;224.502;299.8224]  InternalRulePriority=Speed  RndMeth=Simplest
  To S1 SSL on L5 : PMIOPort  Side=Left
  To L5 SSL on S1 : PMIOPort  Port=2  Side=Left
  To L4 SSL on L5 : PMIOPort  Port=3  Side=Left
  To L5 SSL on L4 : PMIOPort  Port=4  Side=Left
  To L3 SSL on L4 : PMIOPort  Port=5  Side=Left
  To L4 SSL on L3 : PMIOPort  Port=6  Side=Left
  To L2 SSL on L3 : PMIOPort  Port=7  Side=Left
  To L3 SSL on L2 : PMIOPort  Port=8  Side=Left
  To L1 SSL on L2 : PMIOPort  Port=9  Side=Left
  To L2 SSL on L1 : PMIOPort  Port=10  Side=Left
  To ground : PMIOPort  Port=11  Side=Right
  wires:
  Gain2/1 -> Display2/1
  Gain1/1 -> Display1/1
  Gain/1 -> Display/1
  PS-Simulink Converter1/1 -> Gain/1
  PS-Simulink Converter3/1 -> Gain2/1
  PS-Simulink Converter2/1 -> Gain1/1
  Multiply14/1 -> Scope/1, Simulink-PS Converter8/1  "L1-L2 SSL"
  full nonlinear combined4/1 -> Multiply14/1
  Multiply13/1 -> Scope/2, Simulink-PS Converter7/1  "L2-L3 SSL"
  full nonlinear combined3/1 -> Multiply13/1
  Multiply12/1 -> Scope/3, Simulink-PS Converter6/1  "L3-L4 SSL"
  full nonlinear combined2/1 -> Multiply12/1
  Add5/1 -> 2-D Lookup Table2/1, full nonlinear combined2/1
  Multiply11/1 -> Scope/4, Simulink-PS Converter5/1  "L4-L5 SL"
  Add4/1 -> 2-D Lookup Table1/1, full nonlinear combined1/1
  full nonlinear combined1/1 -> Multiply11/1
  Multiply10/1 -> Simulink-PS Converter/1, Scope/5  "L5-S1 SSL"
  full nonlinear combined/1 -> Multiply10/1
  Add3/1 -> bilinear/1, full nonlinear combined/1
  Constant/1 -> Add3/2  "original length"
  PS-Simulink Converter7/1 -> Multiply4/1
  Multiply4/1 -> Add5/1
  PS-Simulink Converter6/1 -> Multiply2/1
  2-D Lookup Table1/1 -> Multiply3/1
  Constant8/1 -> Add7/2
  Constant7/1 -> Add6/2
  PS-Simulink Converter8/1 -> Multiply6/1
  Add7/1 -> 2-D Lookup Table4/1, full nonlinear combined4/1
  Multiply2/1 -> Add4/1
  2-D Lookup Table4/1 -> Multiply9/1
  bilinear/1 -> Multiply1/1
  PS-Simulink Converter/1 -> Multiply/1
  Constant5/1 -> Add4/2
  2-D Lookup Table2/1 -> Multiply5/1
  Multiply6/1 -> Add6/1
  2-D Lookup Table3/1 -> Multiply7/1
  Multiply8/1 -> Add7/1
  Multiply/1 -> Add3/1
  PS-Simulink Converter10/1 -> Multiply8/1
  Add6/1 -> 2-D Lookup Table3/1, full nonlinear combined3/1
  Constant6/1 -> Add5/2
  connections:
  Transform Sensor5/RConn4 -- PS-Simulink Converter3/LConn1
  Transform Sensor5/RConn3 -- PS-Simulink Converter2/LConn1
  Transform Sensor5/RConn2 -- PS-Simulink Converter1/LConn1
  Transform Sensor5/LConn1 -- SSL Visualization/LConn1 -- To ground/RConn1
  Simulink-PS Converter6/RConn1 -- L3-L4 SSL/LConn2
  Simulink-PS Converter5/RConn1 -- L4-L5 SSL/LConn2
  Simulink-PS Converter7/RConn1 -- L2-L3 SSL/LConn2
  L3-L4 SSL/RConn1 -- To L4 SSL on L3/RConn1 -- Visualization/LConn7 -- SSL Visualization/RConn6 -- Transform Sensor2/RConn1
  Transform Sensor3/LConn1 -- SSL Visualization/RConn3 -- To L2 SSL on L3/RConn1 -- Visualization/LConn4 -- L2-L3 SSL/LConn1
  To L2 SSL on L1/RConn1 -- Visualization/LConn10 -- Transform Sensor4/RConn1 -- SSL Visualization/RConn2 -- L1-L2 SSL/RConn1
  PS-Simulink Converter7/LConn1 -- Transform Sensor2/RConn2
  Visualization/LConn6 -- To L3 SSL on L2/RConn1 -- Transform Sensor3/RConn1 -- SSL Visualization/RConn1 -- L2-L3 SSL/RConn1
  PS-Simulink Converter10/LConn1 -- Transform Sensor4/RConn2
  PS-Simulink Converter8/LConn1 -- Transform Sensor3/RConn2
  Transform Sensor2/LConn1 -- SSL Visualization/RConn8 -- Visualization/LConn2 -- To L3 SSL on L4/RConn1 -- L3-L4 SSL/LConn1
  To S1 SSL on L5/RConn1 -- Visualization/LConn9 -- Transform Sensor/RConn1 -- SSL Visualization/RConn9 -- L5-S1 SSL/RConn1
  PS-Simulink Converter/LConn1 -- Transform Sensor/RConn2
  To L5 SSL on L4/RConn1 -- Visualization/LConn8 -- Transform Sensor1/RConn1 -- SSL Visualization/RConn5 -- L4-L5 SSL/RConn1
  PS-Simulink Converter6/LConn1 -- Transform Sensor1/RConn2
  Simulink-PS Converter/RConn1 -- L5-S1 SSL/LConn2
  Transform Sensor4/LConn1 -- SSL Visualization/RConn4 -- To L1 SSL on L2/RConn1 -- Visualization/LConn1 -- L1-L2 SSL/LConn1
  Visualization/LConn3 -- To L4 SSL on L5/RConn1 -- Transform Sensor1/LConn1 -- SSL Visualization/RConn7 -- L4-L5 SSL/LConn1
  Simulink-PS Converter8/RConn1 -- L1-L2 SSL/LConn2
  Transform Sensor/LConn1 -- SSL Visualization/RConn10 -- Visualization/LConn5 -- Transform Sensor5/RConn1 -- To L5 SSL on S1/RConn1 -- L5-S1 SSL/LConn1
